simulink model "ParachuteSpatial3DOF_model"  (R2023b)
settings: Solver=VariableStepAuto  StartTime=0.0  StopTime=100  RelTol=1e-3
model workspace (MAT data in the model file):
  Attachment_Offset_CG = [-20 0 0]
  Cd = 0.8
  Gravity = [0 0 9.81]
  I = [0.210329619662  0  0; 0  130.110649456  0; 0  0  130.110649456]
  Initial_Position = [100 500 10000]
  Initial_Rotation_Offset = [0 3.14159265359 0]
  Initial_Velocity = [0 2 -70]
  Mass = 20
  Parachute_Radius = 1.22
  w0_BN = [0 0 0]
libraries: sharedtransform x3, simulink_extras x2, aerolibanim x1
settings Model: Creator=ben60  LastModifiedBy=thatf
settings ModelReferenceCC: EnableRefExpFcnMdlSchedulingChecks=on

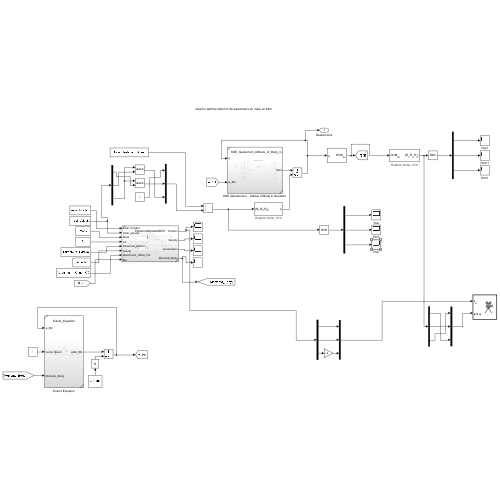
[thumbnail: Simulink's stored preview of the top-level diagram]
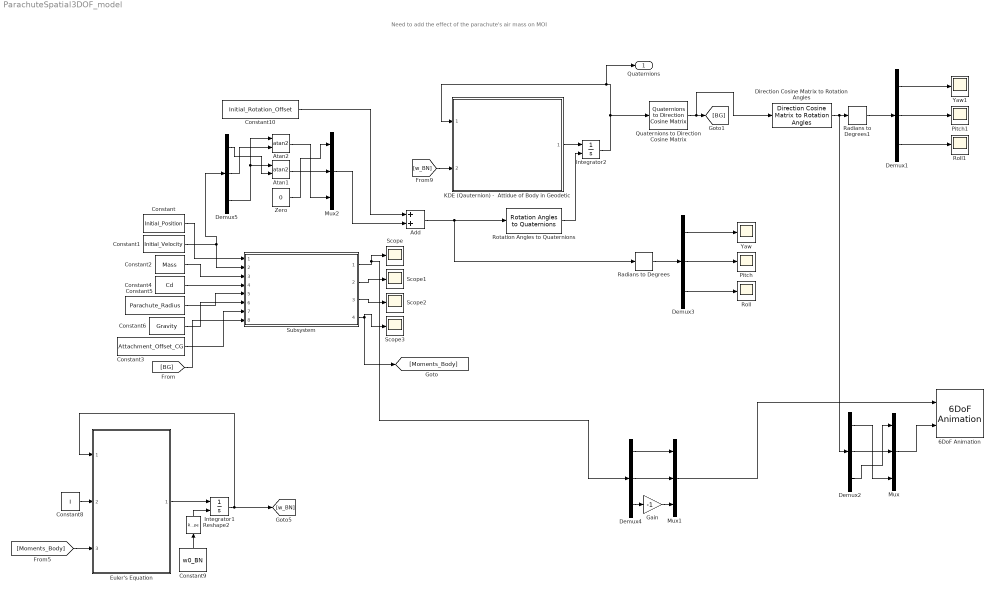
== system ParachuteSpatial3DOF_model ==
  note: Need to add the effect of the parachute's air mass on MOI
  6DoF Animation : aerolibanim/6DoF Animation  u1=[-10 10 -10 10 -10 10]  u2=0.1  u3=1.0  u4=[0 0 0]  u5=Fly alongside  u6=[5 0 0]  u7=10  u8=on
  Add : Sum
  Atan1 : Trigonometry  Operator=atan2
  Atan2 : Trigonometry  Operator=atan2
  Constant : Constant  Value=Initial_Position
  Constant1 : Constant  Value=Initial_Velocity
  Constant10 : Constant  Value=Initial_Rotation_Offset
  Constant2 : Constant  Value=Mass
  Constant3 : Constant  Value=Attachment_Offset_CG
  Constant4 : Constant  Value=Cd
  Constant5 : Constant  Value=Parachute_Radius
  Constant6 : Constant  Value=Gravity
  Constant8 : Constant  Value=I
  Constant9 : Constant  Value=w0_BN
  Demux{1..5} (5 alike) : Demux  Outputs=3
  Direction Cosine Matrix to Rotation Angles : sharedtransform/Direction Cosine Matrix to Rotation Angles  rotationOrder=ZYX  aMode=aMode  action=None  tolerance=eps(2)
  Euler's Equation : Subsystem  ReferencedSubsystem=Eulers_Equation
  Gain : Gain  Gain=-1
  Integrator1 : Integrator  InitialConditionSource=external
  Integrator2 : Integrator  InitialConditionSource=external
  "KDE (Qauternion) -  Attidue of Body in Geodetic " : Subsystem  ReferencedSubsystem=KDE_Qauternion_Attitude_of_Body_in_Geodetic
  Mux : Mux  Inputs=3
  Mux1 : Mux  Inputs=3
  Mux2 : Mux  Inputs=3
  Pitch : Scope
  Pitch1 : Scope
  Quaternions to Direction Cosine Matrix : sharedtransform/Quaternions to  Direction Cosine Matrix  aMode=aMode
  Radians to Degrees : simulink_extras/Transformations/Radians to Degrees
  Radians to Degrees1 : simulink_extras/Transformations/Radians to Degrees
  Reshape2 : Reshape  OutputDimensionality=Customize  OutputDimensions=[3,1]
  Roll : Scope
  Roll1 : Scope
  Rotation Angles to Quaternions : sharedtransform/Rotation Angles to Quaternions  rotationOrder=ZYX  aMode=aMode
  Scope{,1..3} (4 alike) : Scope
  Subsystem : Subsystem  ReferencedSubsystem=ParachuteSpatial3DOF
  Yaw : Scope
  Yaw1 : Scope
  Zero : Constant  Value=0  OutDataTypeStr=Inherit: Inherit via back propagation
  Quaternions : Outport
  wires:
  Subsystem/2 -> Scope1/1
  Subsystem/3 -> Scope2/1
  Constant/1 -> Subsystem/1
  Constant1/1 -> Demux5/1, Subsystem/2
  Constant2/1 -> Subsystem/3
  Constant4/1 -> Subsystem/4
  Constant5/1 -> Subsystem/5
  Constant6/1 -> Subsystem/6
  Subsystem/4 -> Scope3/1, [Moments_Body]
  Constant3/1 -> Subsystem/7
  [BG] -> Subsystem/8
  Constant8/1 -> Euler's Equation/2
  Integrator1/1 -> [w_BN], Euler's Equation/1
  Euler's Equation/1 -> Integrator1/1
  [Moments_Body] -> Euler's Equation/3
  Reshape2/1 -> Integrator1/2
  Constant9/1 -> Reshape2/1
  Demux3/1 -> Yaw/1
  Demux3/2 -> Pitch/1
  Radians to Degrees/1 -> Demux3/1
  Demux3/3 -> Roll/1
  Quaternions to Direction Cosine Matrix/1 -> Direction Cosine Matrix to Rotation Angles/1, [BG]
  Rotation Angles to Quaternions/1 -> Integrator2/2
  "KDE (Qauternion) -  Attidue of Body in Geodetic "/1 -> Integrator2/1
  [w_BN] -> "KDE (Qauternion) -  Attidue of Body in Geodetic "/2
  Integrator2/1 -> Quaternions/1, "KDE (Qauternion) -  Attidue of Body in Geodetic "/1, Quaternions to Direction Cosine Matrix/1
  Demux1/1 -> Yaw1/1
  Radians to Degrees1/1 -> Demux1/1
  Demux1/2 -> Pitch1/1
  Demux1/3 -> Roll1/1
  Demux2/3 -> Mux/1
  Demux2/2 -> Mux/2
  Direction Cosine Matrix to Rotation Angles/1 -> Demux2/1, Radians to Degrees1/1
  Demux2/1 -> Mux/3
  Demux4/3 -> Gain/1
  Gain/1 -> Mux1/3
  Demux4/2 -> Mux1/2
  Demux4/1 -> Mux1/1
  Mux1/1 -> 6DoF Animation/1
  Mux/1 -> 6DoF Animation/2
  Subsystem/1 -> Demux4/1, Scope/1
  Add/1 -> Radians to Degrees/1, Rotation Angles to Quaternions/1
  Constant10/1 -> Add/1
  Mux2/1 -> Add/2
  Atan1/1 -> Mux2/2
  Demux5/3 -> Atan1/1, Atan2/1
  Demux5/2 -> Atan2/2
  Demux5/1 -> Atan1/2
  Atan2/1 -> Mux2/3
  Zero/1 -> Mux2/1
